simulink model "HevP2PowertrainController"  (R2020a)
settings: Solver=FixedStepDiscrete  StartTime=0  StopTime=inf  FixedStep=0.01  RelTol=1e-3  EnableMultiTasking=on
model workspace (MAT data in the model file):
  BattChargeMax = 5.3
  BattChrgPwrMax = -30000
  BattDischrgPwrMax = 46000
  BattEnrgy = 5724000
  BrkPrsMax = 8300000
  CSChrgFctr = 0.2337
  ChrgLmt_bpt = [1 1 1 1 1 1 1 1 0.7 0.35 0]
  DischrgLmt_bpt = [0 0.35 0.7 1 1 1 1 1 1 1 1]
  EVSpdLmt = 17.9
  EngIdle = 78.5398163397
  EngPwr = [1000 7500 15052.6315789 19736.8421053 24421.0526316 29105.2631579 33789.4736842 38473.6842105 43157.8947368 47842.1052632 52526.3157895 57210.5263158 ... (19 elements, 1x19)]
  EngPwr_min = 11408
  EngSpd = [1000 1200 1448.84862461 1712.99052669 1980.33600187 2249.1155588 2517.55970613 2783.89895252 3046.3638066 3303.18477703 3552.59237246 3792.81710154 ... (19 elements, 1x19)]
  EngSpdStart = 20
  EngTrq = [9.54929658551 59.6831036595 99.2112225513 110.02568665 117.759751017 123.57514891 128.166058939 131.971967205 135.285068696 138.308475993 141.18967656 144.040766791 ... (19 elements, 1x19)]
  MotTrq = [200 200 200 200 190.9859317 143.2394488 114.591559 95.49296586 81.85111359 71.61972439 63.66197724 57.29577951 ... (14 elements, 1x14)]
  N = [1 4.212 2.637 1.8 1.386 1 0.772]
  Ndiff = 3.32
  RegenBrkCutOff = [0 1]
  RegenBrkSpd_bpt = [5 9]
  Rm = 0.15
  SOCChrgFctr = 17969
  SOCChrgFctr_SOC_bpt = [50 60]
  SOCChrgFctr_VehSpd_bpt = [2.2352 10]
  SOCTrgt = 60
  SOC_bpt = [0 10 20 30 40 50 60 70 80 90 100]
  SOCmin = 50
  T_eff_bp = [0 20 40 60 80 100 120 140 160 180 200]
  VehMass = 1623
  disk_abore = 0.05
  efficiency_table = [52 52 52 52 52 52 52 52 52 62 66 70 ... (154 elements, 14x11)]
  mu_kinetic = 0.35
  num_pads = 2
  w_eff_bp = [0 500 1000 1432.391138 1500 2000 2500 3000 3500 4000 4500 5000 ... (14 elements, 1x14)]
libraries: simulink x14, autolibutils x2
(part 2 of 2)

== stateflow chart HevP2PowertrainController/P2 Supervisory Control ==
  state Operating_Modes [parallel]
    during:
    PwrCmd = TrqCmd*MotSpd;  % Total Pwr Cmd of actuators at pre-transmission location
    SOCopt = (SOCTrgt/100) - 0.5*VehMass*VehSpd*VehSpd*CSChrgFctr/BattEnrgy;
    ChrgPwr = -SOCChrgFctr*(SOCopt - SOC/100); % negative means Charging needed
    settings: executionOrder=1
    state Driving
      during:
      EngOnReq = EngOnCalc_Drive(BattPwr,BattPwrDischrgLmt,PwrCmd,ChrgPwr,BattPwrChrgLmt);
      state EV
        entry, during:
        OpMode = 1;
      state PHEV
        entry, during:
        OpMode = 3;
        [MotPwrCmd,EngPwrCmd] = PHEV(TrqCmd,MotSpd,PwrCmd,EngTrqOut,ChrgPwr,BattPwrChrgLmt,BattPwrDischrgLmt);
        exit:
        EngPwrCmd = 0;
        MotPwrCmd = 0;
        state [MotPwrCmd,EngPwrCmd] = PHEV(TrqCmd,MotSpd,PwrCmd,EngTrqOut,ChrgPwr,BattPwrChrgLmt,BattPwrDischrgLmt) [function]
      state Wait
        entry, during:
        OpMode = 2;
      state EngOnReq = EngOnCalc_Drive(BattPwr,BattPwrDischrgLmt,PwrCmd,ChrgPwr,BattPwrChrgLmt) [function]
      (default) -> EV
      EV -> Wait : [EngOnReq]
      Wait -> Operating_Modes.Driving.PHEV [order 1] : [EngStarted]
      Wait -> EV [order 2] : [~EngOnReq]
      Operating_Modes.Driving.PHEV -> EV : [~EngOnReq]
    state Stationary_Charging
      entry, during:
      Park = 1;
      Neutral = 1;
      EngOnReq = ...
      EngOnCalc_Stationary(SOC);
      exit:
      Park = 0;
      Neutral = 0;
      state Off
        entry, during:
        OpMode = 7;
      state Eng_Start
        entry, during:
        OpMode = 8;
      state Charging
        entry, during:
        OpMode = 9;
        EngPwrCmd = ChargePowerCalc(BattPwrChrgLmt);
        exit:
        EngPwrCmd = 0;
        state EngPwrCmd = ChargePowerCalc(BattPwrChrgLmt) [function]
      state Eng_Brake
        entry, during:
        OpMode = 10;
      state EngOnReq = EngOnCalc_Stationary(SOC) [function]
      (default) -> Operating_Modes.Stationary_Charging.Off
      Operating_Modes.Stationary_Charging.Off -> Eng_Start [order 2] : [EngOnReq ...
          | && TransGear == 0]
      Eng_Start -> Charging : [EngStarted]
      Charging -> Eng_Brake : [~EngOnReq]
      Eng_Brake -> Operating_Modes.Stationary_Charging.Off : [EngSpd < 1]
    (default) -> Operating_Modes.Driving
    Operating_Modes.Driving -> Operating_Modes.Stationary_Charging : [Chrg]
    Operating_Modes.Stationary_Charging.Off -> Operating_Modes.Driving [order 1] : [~Chrg]
  state Motor_Control [parallel]
    settings: executionOrder=2
    state TractionModes
      state Mot_EV
        entry, during:
        MotTrqCmd = MotTrqEV(TrqCmd);
        MotMode = 1;
        state MotTrqCmd = MotTrqEV(TrqCmd) [function]
      state Mot_PHEV
        entry, during:
        MotTrqCmd = MotTrqHEV(MotPwrCmd,MotSpd);
        MotMode = 2;
        state MotTrqCmd = MotTrqHEV(MotPwrCmd,MotSpd) [function]
      (default) -> Mot_EV
      Mot_PHEV -> Mot_EV : [OpMode == 1 ...
          |  || OpMode == 2]
      Mot_EV -> Mot_PHEV : [OpMode == 3]
    state Mot_ChargingMode
      entry, during:
      MotMode = 3;
      MotTrqCmd = SpdControl(EngSpd,EngSpdCmd);
      state MotTrqCmd = SpdControl(EngSpd,EngSpdCmd) [function]
    (default) -> TractionModes
    TractionModes -> Mot_ChargingMode : [OpMode == 8]
    Mot_ChargingMode -> TractionModes : [OpMode == 7]
  state Engine_Control [parallel]
    settings: executionOrder=3
    state Off
      entry, during:
      EngMode = 1;
      EngTrqCmd = 0;
      EngSpdCmd = 0;
      StartCmd = 0;
      EngStarted = 0;
      Cltch1Cmd = 0;
    state Starting
      state CheckPark
      state Stationary
        state Start
          entry:
          EngMode = 10;
          Cltch1Cmd = 1;
        state LowSOC_Start
          entry:
          EngMode = 9;
          EngTrqCmd = 0;
          EngSpdCmd = 0;
          StartCmd = 1;
          exit:
          StartCmd = 0;
        state MotorStart
          entry:
          EngMode = 2;
          EngTrqCmd = 0;
          EngSpdCmd = EngIdle;
          exit:
          EngSpdCmd = 0;
        (default) -> Engine_Control.Starting.Stationary.Start
        Engine_Control.Starting.Stationary.Start -> (junction 1030) : [Cltch1State && ...
            |  TransGear == 0]
        (junction 1030) -> LowSOC_Start [order 1] : [SOC < SOCmin]
        (junction 1030) -> MotorStart [order 2]
      state Driving
        state Start
          entry, during:
          EngMode = 3;
          EngTrqCmd = 0;
          EngSpdCmd = 0;
          StartCmd = 1;
          exit:
          StartCmd = 0;
        state EngSpdMatch
          entry, during:
          EngMode = 11;
          [EngTrqCmd,CloseCltch] = EngMatch(MotSpd,EngSpd);
          state [EngTrqCmd,CloseCltch] = EngMatch(MotSpd,EngSpd) [function]
        state CloseCltch
          entry, during:
          EngMode = 12;
          EngTrqCmd = 0;
          Cltch1Cmd = 1;
        (default) -> Engine_Control.Starting.Driving.Start
        Engine_Control.Starting.Driving.Start -> EngSpdMatch : [EngSpd > EngSpdStart]
        EngSpdMatch -> CloseCltch : [CloseCltch]
      (default) -> CheckPark
      CheckPark -> (junction 1069) [order 2] : [~Park]
      (junction 1069) -> Engine_Control.Starting.Driving : [~Cltch1State]
      CheckPark -> Stationary [order 1] : [Park]
      Stationary -> (junction 1094) : [EngSpd > EngSpdStart]
      CloseCltch -> (junction 1094) : [EngSpd > EngSpdStart && Cltch1State]
    state On
      en:
      EngStarted = 1;
      state Stationary_Charging
        entry, during:
        EngMode = 4;
        [EngTrqCmd,EngSpdCmd] = EngChrg(EngPwrCmd);
        state [EngTrqCmd,EngSpdCmd] = EngChrg(EngPwrCmd) [function]
      state PHEV
        entry, during:
        EngMode = 5;
        EngTrqCmd = EngPHEV(EngPwrCmd);
        state EngTrqCmd = EngPHEV(EngPwrCmd) [function]
      (default) -> Engine_Control.On.Stationary_Charging
      Engine_Control.On.Stationary_Charging -> Engine_Control.On.PHEV : [~Park]
      Engine_Control.On.PHEV -> Engine_Control.On.Stationary_Charging : [Park && OpMode == 9]
    state EngBrake
      entry, during:
      EngMode = 8;
      EngTrqCmd = 0;
      EngSpdCmd = 0;
    (default) -> Engine_Control.Off
    (junction 1094) -> On
    Engine_Control.Off -> Starting : [EngOnReq]
    Starting -> Engine_Control.Off : [~EngOnReq]
    EngBrake -> Engine_Control.Off : [EngSpd < 1]
    (junction 1116) -> Engine_Control.Off [order 2] : [~Chrg]
    (junction 1116) -> EngBrake [order 1] : [Chrg]
    On -> (junction 1116) : [~EngOnReq]
  data: TrqCmd function_input; MotPwrCmd function_output; MotSpd function_input; PwrCmd function_input; EngTrqOut function_input; EngPwrCmd function_output; ChrgPwr function_input; BattPwrChrgLmt function_input; BattPwrDischrgLmt function_input; EngOnReq function_output; BattPwr function_input; BattPwrDischrgLmt function_input; PwrCmd function_input; ChrgPwr function_input; BattPwrChrgLmt function_input; BattPwrChrgLmt function_input; EngPwrCmd function_output; SOC function_input; EngOnReq function_output; TrqCmd function_input; MotTrqCmd function_output; MotPwrCmd function_input; MotTrqCmd function_output; MotSpd function_input; EngSpd function_input; MotTrqCmd function_output; EngSpdCmd function_input; MotSpd function_input; EngTrqCmd function_output; EngSpd function_input; CloseCltch function_output; EngPwrCmd function_input; EngTrqCmd function_output; EngSpdCmd function_output; EngPwrCmd function_input; EngTrqCmd function_output; EVSpdLmt input; EngIdle input; EngSpdStart input; SOCTrgt input =60; SOCmin input [SOCmin..]; CSChrgFctr input; BattEnrgy input =4717440; VehMass input =1310; SOC input; SOCChrgFctr input =150000; OpMode output double; MotMode output double; EngOnReq output double; EngMode output double; EngPwrCmd output double; MotPwrCmd output double; ChrgPwr output double; PwrCmd output double; SOCopt output double; VehSpd input; MotSpd input; BattPwrDischrgLmt input; BattPwrChrgLmt input; TransGear input; Cltch1State input; Chrg input; Cltch2State input; EngTrqOut input; BattPwr input; EngSpd input; TrqCmd input; EngSpdCmd output double; Park output double; StartCmd output double; Cltch1Cmd output double; Neutral output double; EngTrqCmd output double; MotTrqCmd output double; EngStarted local double; CloseCltch local double

== stateflow chart HevP2PowertrainController/P2 Supervisory Control/Operating_Modes.Driving.EngOnCalc_Drive/Check Power1/Timer ==
  state Wait
    du:
    Out = 0;
  state StartTimer
    du:
    Out = 0;
  state TimerDone
    du:
    Out = 1;
  (default) -> StartTimer
  StartTimer -> Wait : [In]
  Wait -> TimerDone [order 2] : after(1, sec)
  Wait -> StartTimer [order 1] : [~In]
  TimerDone -> StartTimer : [~In && after(1, sec)]
  data: In input; Out output
